simulink model "UT5"  (R2022a)
settings: Solver=FixedStepDiscrete  StartTime=0.0  StopTime=2600000  RelTol=1e-3
values from neighbouring files (symbols this model uses):
  stock = 4.857316332726169e6    (= 4857316.33273)    [Battery.m]
undefined symbols (not defined in the file or in its folder): Breakpoints, hys_max, hys_min, max_soc, min_soc, P_engage, R2_B, R2_H, SimulationStep
libraries: Assets x3, eeGeneralControl x1
settings Model: Creator=a.dehghan  LastModifiedBy=a.dehghan

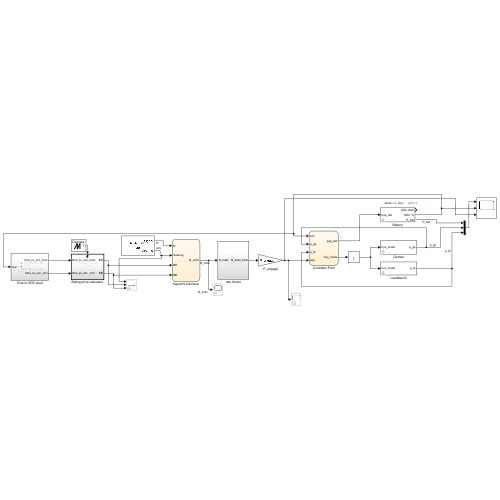
[thumbnail: Simulink's stored preview of the top-level diagram]
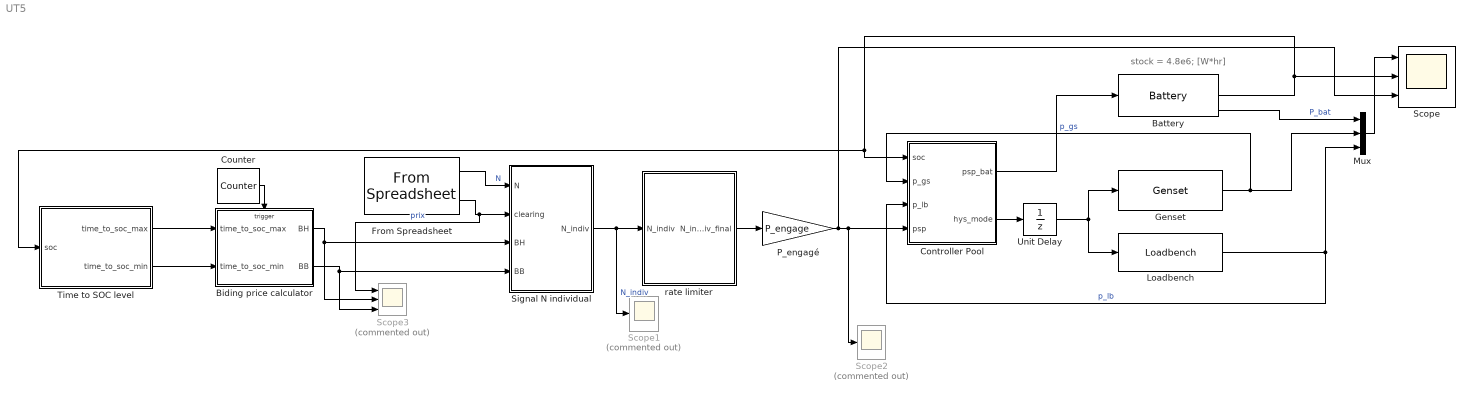
== system UT5 ==
  note: stock = 4.8e6; [W*hr]
  Battery : Assets/Battery  max_soc_limit=max_soc_limit  min_soc_limit=min_soc_limit  efficiency_discharge=efficiency_discharge  efficiency_charge=efficiency_charge  psp_bat=p  stock=stock  ini_state_of_charge=ini_state_of_charge
      settings: SourceProductName=My Library
  Biding price calculator : Subsystem  TreatAsAtomicUnit=on
  Controller Pool : Stateflow chart  TreatAsAtomicUnit=on
  Counter : eeGeneralControl/Counter  CarrCount=Up  Range=[0 1]  Tper=900  Tdelay=0  Ts=1
      settings: SourceProductBaseCode=PS
  From Spreadsheet : FromSpreadsheet  FileName=N_Jan.xlsx  SheetName=30
  Genset : Assets/Genset  hys_mode=[0 -1]  p_max_gs=p_max_gs  rising_slew_rate=rising_slew_rate  falling_slew_rate=falling_slew_rate
      settings: SourceProductName=My Library
  Loadbench : Assets/Loadbench  hys_mode=[0 1]  p_max_lb=p_max_lb
      settings: SourceProductName=My Library
  Mux : Mux  Inputs=3
  P_engagé : Gain  Gain=P_engage
  Scope : Scope  NumInputPorts=3
  Scope1 : Scope  Commented=on
  Scope2 : Scope  Commented=on
  Scope3 : Scope  Commented=on  NumInputPorts=3
  Signal N individual : Stateflow chart  TreatAsAtomicUnit=on
  Time to SOC level : Subsystem
  Unit Delay : UnitDelay  HasFrameUpgradeWarning=on
  rate limiter : Subsystem
  wires:
  From Spreadsheet/1 -> Signal N individual/1(N)  "N"
  P_engagé/1 -> Scope/3, Scope2/1, Controller Pool/4(psp)
  Time to SOC level/1(time_to_soc_max) -> Biding price calculator/1(time_to_soc_max)
  Counter/1 -> Biding price calculator/Trigger
  Biding price calculator/1(BH) -> Scope3/2, Signal N individual/3(BH)
  Time to SOC level/2(time_to_soc_min) -> Biding price calculator/2(time_to_soc_min)
  Biding price calculator/2(BB) -> Signal N individual/4(BB), Scope3/3
  From Spreadsheet/2 -> Scope3/1, Signal N individual/2(clearing)  "prix"
  rate limiter/1(N_indiv_final) -> P_engagé/1
  Mux/1 -> Scope/1
  Genset/1 -> Controller Pool/2(p_gs), Mux/2  "p_gs"
  Controller Pool/2(hys_mode) -> Unit Delay/1
  Unit Delay/1 -> Genset/1, Loadbench/1
  Signal N individual/1(N_indiv) -> Scope1/1, rate limiter/1(N_indiv)  "N_indiv"
  Loadbench/1 -> Controller Pool/3(p_lb), Mux/3  "p_lb"
  Battery/2 -> Scope/2, Time to SOC level/1(soc), Controller Pool/1(soc)
  Controller Pool/1(psp_bat) -> Battery/1
  Battery/3 -> Mux/1  "P_bat"

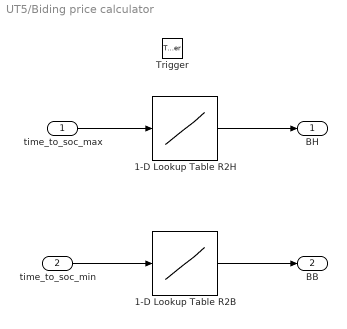
== system UT5/Biding price calculator ==
  time_to_soc_max : Inport
  time_to_soc_min : Inport  Port=2
  Trigger : TriggerPort  VariantControl=(inherit)
  1-D Lookup Table R2B : Lookup_n-D  NumberOfTableDimensions=1  BreakpointsForDimension1=Breakpoints  BeginIndexSearchUsingPreviousIndexResult=on  Table=R2_B  InternalRulePriority=Speed  RndMeth=Simplest
  1-D Lookup Table R2H : Lookup_n-D  NumberOfTableDimensions=1  BreakpointsForDimension1=Breakpoints  BeginIndexSearchUsingPreviousIndexResult=on  Table=R2_H  InternalRulePriority=Speed  RndMeth=Simplest
  BH : Outport
  BB : Outport  Port=2
  wires:
  time_to_soc_max/1 -> 1-D Lookup Table R2H/1
  1-D Lookup Table R2H/1 -> BH/1
  time_to_soc_min/1 -> 1-D Lookup Table R2B/1
  1-D Lookup Table R2B/1 -> BB/1

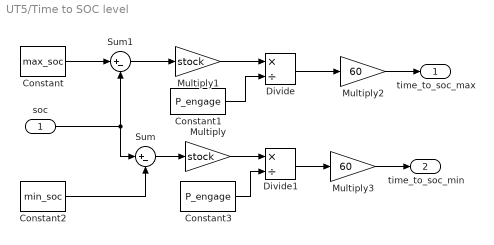
== system UT5/Time to SOC level ==
  soc : Inport
  Constant : Constant  Value=max_soc
  Constant1 : Constant  Value=P_engage
  Constant2 : Constant  Value=min_soc
  Constant3 : Constant  Value=P_engage
  Divide : Product  Inputs=*/
  Divide1 : Product  Inputs=*/
  Multiply : Gain  Gain=stock
  Multiply1 : Gain  Gain=stock
  Multiply2 : Gain  Gain=60
  Multiply3 : Gain  Gain=60
  Sum : Sum  Inputs=|+-
  Sum1 : Sum  Inputs=|+-
  time_to_soc_max : Outport
  time_to_soc_min : Outport  Port=2
  wires:
  Sum/1 -> Multiply/1
  Constant2/1 -> Sum/2
  soc/1 -> Sum1/2, Sum/1
  Constant/1 -> Sum1/1
  Sum1/1 -> Multiply1/1
  Multiply/1 -> Divide1/1
  Multiply1/1 -> Divide/1
  Constant1/1 -> Divide/2
  Constant3/1 -> Divide1/2
  Divide1/1 -> Multiply3/1
  Divide/1 -> Multiply2/1
  Multiply2/1 -> time_to_soc_max/1
  Multiply3/1 -> time_to_soc_min/1

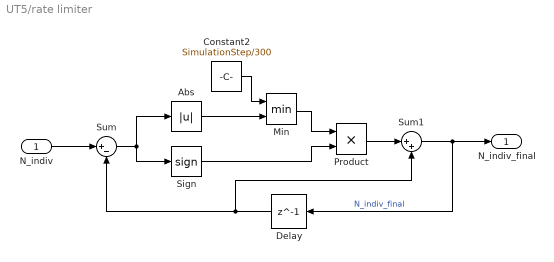
== system UT5/rate limiter ==
  N_indiv : Inport
  Abs : Abs  SaturateOnIntegerOverflow=off
  Constant2 : Constant  Value=SimulationStep/300
  Delay : Delay  DelayLength=1
  Min : MinMax  Inputs=2
  Product : Product
  Sign : Signum
  Sum : Sum  Inputs=|+-
  Sum1 : Sum  Inputs=|++
  N_indiv_final : Outport
  wires:
  Sum/1 -> Sign/1, Abs/1
  Delay/1 -> Sum/2, Sum1/2
  Product/1 -> Sum1/1
  Min/1 -> Product/1
  Sum1/1 -> Delay/1, N_indiv_final/1  "N_indiv_final"
  Sign/1 -> Product/2
  Abs/1 -> Min/2
  Constant2/1 -> Min/1
  N_indiv/1 -> Sum/1

== stateflow chart UT5/Controller Pool ==
  state ? [commented out]
    state Battery1 [commented out]
      entry : p_cons = psp_bat;
      during :
      psp_gs = 0;
      psp_lb = 0;
    state Genset1 [commented out]
      entry : p_cons = psp_gs;
      during :
      psp_lb = 0;
      psp_bat = 0;
    state Loadbench1 [commented out]
      entry : p_cons = psp_lb
      during :
      psp_gs = 0;
      psp_bat = 0;
    ?.Battery1 -> Genset1 [commented out] : [SOC < min_soc && p_cons >=0]
    Genset1 -> ?.Battery1 [commented out] : [min_soc < SOC < max_soc]
    Genset1 -> Loadbench1 [commented out] : [SOC > max_soc && p_cons <=0]
    Loadbench1 -> Genset1 [commented out]
    Loadbench1 -> ?.Battery1 [commented out] : [min_soc < SOC < max_soc]
    ?.Battery1 -> Loadbench1 [commented out]
  state Hysteresis_mode
    state Mode___1
      en : hys_mode = -1;
      du : psp_bat = psp - p_lb - p_gs;
    state Mode_0
      en : hys_mode = 0;
      du : psp_bat = psp - p_lb - p_gs;
    state Mode_1
      en : hys_mode = 1;
      du : psp_bat = psp - p_lb - p_gs;
    (default) -> Mode_0
    Mode_0 -> Mode___1 [order 2] : [soc <= min_soc]
    Mode_0 -> Mode_1 [order 1] : [soc >= max_soc]
    Mode___1 -> Mode_0 : [soc >= hys_min]
    Mode_1 -> Mode_0 : [soc <= hys_max]
  state Dispatcher1 [commented out]
    state Battery1 [commented out]
      en :
      hys_mode = 0;
      p_cons = psp_bat;
    state LB_off [commented out]
      en : hys_mode = 0;
      du : p_cons = psp_bat;
    state LB_on [commented out]
      en : hys_mode = 1;
      du : p_cons = psp_lb;
    state GS_on [commented out]
      en : hys_mode = -1;
      du : p_cons = psp_gs;
    state GS_off [commented out]
      en : hys_mode = 0;
      du : p_cons = psp_bat;
    (default) -> Dispatcher1.Battery1 [commented out]
    Dispatcher1.Battery1 -> (junction 131) [commented out]
    (junction 131) -> GS_off [commented out] : [soc >= hys_min]
    (junction 131) -> LB_on [commented out] : [soc >= hys_max]
    (junction 131) -> GS_on [commented out] : [soc <= hys_min]
    (junction 131) -> LB_off [commented out] : [soc <= hys_max]
  state start_order [commented out]
    (default) -> (junction 74) [commented out] : % start_order
    (junction 74) -> (junction 75) [commented out] : [psp_gs > 0]
    (junction 74) -> (junction 76) [commented out] : {start_order = 0;}
    (junction 75) -> (junction 77) [commented out] : {start_order = 1;}
    (junction 77) -> (junction 76) [commented out]
    (junction 76) -> (junction 78) [commented out]
  state ? [commented out]
    state Battery [commented out]
      entry : p_cons = psp_bat;
      during :
      psp_gs = 0;
      psp_lb = 0;
    state Genset [commented out]
      entry : p_cons = psp_gs;
      during :
      psp_lb = 0;
      psp_bat = 0;
    state Loadbench [commented out]
      entry : p_cons = psp_lb
      during :
      psp_gs = 0;
      psp_bat = 0;
    (default) -> (junction 91) [commented out]
    (junction 91) -> Genset [commented out] : [SOC < min_soc && p_cons >=0]
    (junction 91) -> Loadbench [commented out] : [SOC > max_soc && p_cons <=0]
    (junction 91) -> Battery [commented out]
  data: soc input; p_gs input; p_lb input; psp_bat output; hys_mode output; psp input; min_soc parameter double; max_soc parameter double; hys_max parameter; hys_min parameter

== stateflow chart UT5/Signal N individual ==
  state Baisse
    en :  N_indiv = -1;
  state N_0
    en : N_indiv = 0;
  state Hausse
    en : N_indiv = 1;
  (default) -> N_0
  Baisse -> N_0 : [clearing > BB]
  N_0 -> Hausse [order 1] : [clearing >= BH && N >0 ]
  N_0 -> Baisse [order 2] : [clearing <= BB && N <0]
  Hausse -> N_0 : [clearing < BH]
  data: N input; clearing input; BH input; BB input; N_indiv output
